simulink model "ModBateria"  (R2023a)
settings: Solver=VariableStepAuto  StartTime=0.0  StopTime=3600  RelTol=1e-3  AbsTol=1e-3  EnableMultiTasking=on
libraries: fl_lib x6, nesl_utility x5, batteryecm_lib x1
settings Model: Creator=Julian  LastModifiedBy=Julian
settings SolverCC: AutoScaleAbsTol=off  AlgebraicLoopSolver=TrustRegion  MaxZcPerStep=1
settings DataIOCC: LimitDataPoints=on  MaxDataPoints=10000
settings OptimizationCC: ReuseModelBlockBuffer=off  LifeSpan=inf
settings DebuggingCC: UnconnectedInputMsg=warning  UnconnectedOutputMsg=warning  UnconnectedLineMsg=warning  AllowSymbolicDim=off  SFUnexpectedBacktrackingDiag=warning  SFNoUnconditionalDefaultTransitionDiag=warning  SFExecutionAtInitializationDiag=none  ArithmeticOperatorsInVariantConditions=warning
settings ModelReferenceCC: EnableRefExpFcnMdlSchedulingChecks=on
settings SFSimCC: SimUseLocalCustomCode=off  CustomCodeUndefinedFunction=UseInterfaceOnly
settings RTWCC: RTWUseLocalCustomCode=off  DLArmComputeVersion=19.05
settings CodeAppCC: StateflowObjectComments=on
settings GRTTargetCC: TargetLangStandard=C89/C90 (ANSI)
settings ConfigComp: CovMetricSettings=dw  CovSaveCumulativeToWorkspaceVar=on  CovSaveSingleToWorkspaceVar=on  CovExternalEMLEnable=off  CovSFcnEnable=off
settings SimscapeCC: SimscapeLogType=all  SimscapeLogSimulationStatistics=on  SimscapeLogDataHistory=10000

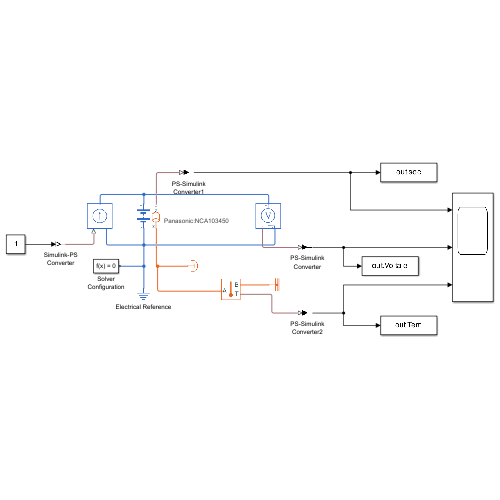
[thumbnail: Simulink's stored preview of the top-level diagram]
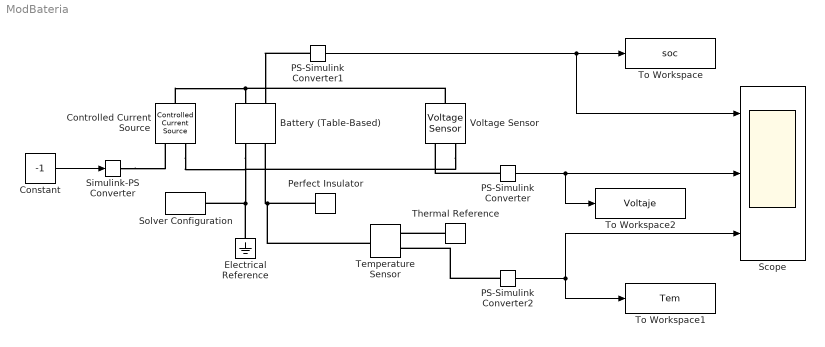
== system ModBateria ==
  Battery (Table-Based) : batteryecm_lib/Battery (Table-Based)  Tag={'toolbox/physmod/battery/shared_library/m/batteryecm_lib_parts';'Battery__Table_Based_/Panasonic/NCA103450.xml'}  SOC_vec=[0 0.01 0.02 0.03 0.04 0.05 0.06 0.07 0.08 0.09 0.1 0.11 0.12 0.13 0.14 0.15 0.16 0.17 0.18 0.19 0.2 0.21 0.22 0.23 0.24 0.25 0.26 0.27 0.28 0.29 0.3 0.31 0.32 0.33 0.34 0.35 0.36 0.37 0.38 0.39 0.4 0.41 0.42 0.43 0.44 0.45 0.46 0.47 0.48 0.49 0.5 0.51 0.52 0.53 0.54 0.55 0.56 0.57 0.58 0.59 0.6 0.61 0.62 0.63 0.64 0.65 0.66 0.67 0.68 0.69 0.7 0.71 0.72 0.73 0.74 0.75 0.76 0.77 0.78 0.79 0.8 0.81 0.82 0.83 0.84 0.85 0.86 0.87 0.88 0.89 0.9 0.91 0.92 0.93 0.94 0.95 0.96 0.97 0.98 0.99 1]  T_dependence=simscape.enum.tablebattery.temperature_dependence.yes  prm_dir=simscape.enum.tablebattery.prm_dir.noCurrentDirectionality  T_vec=[-20 -10 0 25 40] degC  V0_mat=[2.78866 2.78866 2.78866 2.78866 2.78866;2.85705 2.85705 2.85705 2.85705 2.85705;2.9399 2.9399 2.9399 2.9399 2.9399;2.9762 2.9762 2.9762 2.9762 2.9762;3.01251 3.01251 3.01251 3.01251 3.01251;3.04882 3.04882 3.04882 3.04882 3.04882;3.10085 3.10085 3.10085 3.10085 3.10085;3.15288 3.15288 3.15288 3.15288 3.15288;3.19526 3.19526 3.19526 3.19526 3.19526;3.23378 3.23378 3.23378 3.23378 3.23378;3.27026 3.27026 3.27026 3.27026 3.27026;3.29683 3.29683 3.29683 3.29683 3.29683;3.3202 3.3202 3.3202 3.3202 3.3202;3.34216 3.34216 3.34216 3.34216 3.34216;3.36071 3.36071 3.36071 3.36071 3.36071;3.37869 3.37869 3.37869 3.37869 3.37869;3.39522 3.39522 3.39522 3.39522 3.39522;3.40936 3.40936 3.40936 3.40936 3.40936;3.42116 3.42116 3.42116 3.42116 3.42116;3.43247 3.43247 3.43247 3.43247 3.43247;3.44296 3.44296 3.44296 3.44296 3.44296;3.45253 3.45253 3.45253 3.45253 3.45253;3.4621 3.4621 3.4621 3.4621 3.4621;3.47168 3.47168 3.47168 3.47168 3.47168;3.47981 3.47981 3.47981 3.47981 3.47981;3.48589 3.48589 3.48589 3.48589 3.48589;3.49191 3.49191 3.49191 3.49191 3.49191;3.49852 3.49852 3.49852 3.49852 3.49852;3.50514 3.50514 3.50514 3.50514 3.50514;3.51166 3.51166 3.51166 3.51166 3.51166;3.51793 3.51793 3.51793 3.51793 3.51793;3.52413 3.52413 3.52413 3.52413 3.52413;3.53014 3.53014 3.53014 3.53014 3.53014;3.5361 3.5361 3.5361 3.5361 3.5361;3.5422 3.5422 3.5422 3.5422 3.5422;3.5486 3.5486 3.5486 3.5486 3.5486;3.55501 3.55501 3.55501 3.55501 3.55501;3.56135 3.56135 3.56135 3.56135 3.56135;3.56757 3.56757 3.56757 3.56757 3.56757;3.57378 3.57378 3.57378 3.57378 3.57378;3.5802 3.5802 3.5802 3.5802 3.5802;3.58658 3.58658 3.58658 3.58658 3.58658;3.59285 3.59285 3.59285 3.59285 3.59285;3.59911 3.59911 3.59911 3.59911 3.59911;3.60522 3.60522 3.60522 3.60522 3.60522;3.61126 3.61126 3.61126 3.61126 3.61126;3.6173 3.6173 3.6173 3.6173 3.6173;3.62334 3.62334 3.62334 3.62334 3.62334;3.62937 3.62937 3.62937 3.62937 3.62937;3.63541 3.63541 3.63541 3.63541 3.63541;3.64172 3.64172 3.64172 3.64172 3.64172;3.65002 3.65002 3.65002 3.65002 3.65002;3.65922 3.65922 3.65922 3.65922 3.65922;3.66843 3.66843 3.66843 3.66843 3.66843;3.67774 3.67774 3.67774 3.67774 3.67774;3.68705 3.68705 3.68705 3.68705 3.68705;3.69636 3.69636 3.69636 3.69636 3.69636;3.70567 3.70567 3.70567 3.70567 3.70567;3.71498 3.71498 3.71498 3.71498 3.71498;3.72395 3.72395 3.72395 3.72395 3.72395;3.73263 3.73263 3.73263 3.73263 3.73263;3.74129 3.74129 3.74129 3.74129 3.74129;3.74974 3.74974 3.74974 3.74974 3.74974;3.75815 3.75815 3.75815 3.75815 3.75815;3.76656 3.76656 3.76656 3.76656 3.76656;3.77497 3.77497 3.77497 3.77497 3.77497;3.78345 3.78345 3.78345 3.78345 3.78345;3.79201 3.79201 3.79201 3.79201 3.79201;3.80058 3.80058 3.80058 3.80058 3.80058;3.80915 3.80915 3.80915 3.80915 3.80915;3.81772 3.81772 3.81772 3.81772 3.81772;3.8263 3.8263 3.8263 3.8263 3.8263;3.83493 3.83493 3.83493 3.83493 3.83493;3.84366 3.84366 3.84366 3.84366 3.84366;3.8525 3.8525 3.8525 3.8525 3.8525;3.86255 3.86255 3.86255 3.86255 3.86255;3.87289 3.87289 3.87289 3.87289 3.87289;3.88332 3.88332 3.88332 3.88332 3.88332;3.89375 3.89375 3.89375 3.89375 3.89375;3.90419 3.90419 3.90419 3.90419 3.90419;3.91462 3.91462 3.91462 3.91462 3.91462;3.92505 3.92505 3.92505 3.92505 3.92505;3.93549 3.93549 3.93549 3.93549 3.93549;3.9468 3.9468 3.9468 3.9468 3.9468;3.95849 3.95849 3.95849 3.95849 3.95849;3.97034 3.97034 3.97034 3.97034 3.97034;3.98295 3.98295 3.98295 3.98295 3.98295;3.99562 3.99562 3.99562 3.99562 3.99562;4.0083 4.0083 4.0083 4.0083 4.0083;4.02097 4.02097 4.02097 4.02097 4.02097;4.03332 4.03332 4.03332 4.03332 4.03332;4.04495 4.04495 4.04495 4.04495 4.04495;4.05596 4.05596 4.05596 4.05596 4.05596;4.06698 4.06698 4.06698 4.06698 4.06698;4.0778 4.0778 4.0778 4.0778 4.0778;4.0887 4.0887 4.0887 4.0887 4.0887;4.10062 4.10062 4.10062 4.10062 4.10062;4.11408 4.11408 4.11408 4.11408 4.11408;4.12548 4.12548 4.12548 4.12548 4.12548;4.13345 4.13345 4.13345 4.13345 4.13345;4.05294 4.05294 4.05294 4.05294 4.05294] V  V0_vec=[2.78866 2.85705 2.9399 2.9762 3.01251 3.04882 3.10085 3.15288 3.19526 3.23378 3.27026 3.29683 3.3202 3.34216 3.36071 3.37869 3.39522 3.40936 3.42116 3.43247 3.44296 3.45253 3.4621 3.47168 3.47981 3.48589 3.49191 3.49852 3.50514 3.51166 3.51793 3.52413 3.53014 3.5361 3.5422 3.5486 3.55501 3.56135 3.56757 3.57378 3.5802 3.58658 3.59285 3.59911 3.60522 3.61126 3.6173 3.62334 3.62937 3.63541 3.64172 3.65002 3.65922 3.66843 3.67774 3.68705 3.69636 3.70567 3.71498 3.72395 3.73263 3.74129 3.74974 3.75815 3.76656 3.77497 3.78345 3.79201 3.80058 3.80915 3.81772 3.8263 3.83493 3.84366 3.8525 3.86255 3.87289 3.88332 3.89375 3.90419 3.91462 3.92505 3.93549 3.9468 3.95849 3.97034 3.98295 3.99562 4.0083 4.02097 4.03332 4.04495 4.05596 4.06698 4.0778 4.0887 4.10062 4.11408 4.12548 4.13345 4.05294] V  V_range=[2.475 Inf] V  R0_mat=[0.53219 0.30004 0.37039 0.09603 0.02438;0.53219 0.49271 0.49416 0.09983 0.00588;0.53219 0.4834 0.47641 0.10832 0.00588;0.53219 0.47409 0.45867 0.10252 0.00588;0.53219 0.46477 0.44092 0.09675 0.00588;0.53219 0.45546 0.42317 0.09122 0.00588;0.53219 0.44615 0.40543 0.09227 0.01303;0.53219 0.43683 0.38768 0.09475 0.02948;0.53219 0.42752 0.36993 0.09603 0.04205;0.53219 0.4182 0.35219 0.09767 0.05287;0.53219 0.40889 0.33444 0.10033 0.06277;0.53219 0.39958 0.31669 0.10063 0.06815;0.53219 0.39026 0.29895 0.10093 0.07208;0.53219 0.38095 0.2812 0.10152 0.07537;0.53219 0.37164 0.26345 0.10164 0.07711;0.53219 0.36232 0.24546 0.10179 0.0786;0.52242 0.35301 0.22688 0.10206 0.081;0.51265 0.3437 0.2212 0.1018 0.0832;0.50288 0.33438 0.21445 0.10114 0.08432;0.49311 0.32507 0.20748 0.101 0.08523;0.48334 0.31575 0.20014 0.10083 0.08577;0.47357 0.30603 0.19554 0.10046 0.08589;0.4638 0.29631 0.19194 0.1001 0.086;0.45402 0.28659 0.18835 0.09973 0.08612;0.44425 0.27918 0.1841 0.09895 0.08559;0.43448 0.27108 0.17892 0.09787 0.08412;0.42471 0.26296 0.17371 0.09686 0.08262;0.41494 0.2551 0.16877 0.0964 0.08139;0.40517 0.24775 0.16605 0.09595 0.08017;0.3954 0.2429 0.16407 0.09547 0.07932;0.38563 0.23793 0.16198 0.09493 0.07894;0.37586 0.23293 0.15986 0.09438 0.07852;0.36609 0.22784 0.15765 0.09383 0.07801;0.35632 0.22273 0.15542 0.09328 0.07749;0.34661 0.21769 0.15325 0.09286 0.07702;0.33705 0.21414 0.15123 0.09268 0.0767;0.32749 0.2112 0.1492 0.0925 0.07637;0.31951 0.20824 0.14714 0.0923 0.07602;0.31183 0.20521 0.14536 0.09207 0.07561;0.30415 0.20219 0.14439 0.09183 0.0752;0.29737 0.19925 0.1435 0.09158 0.07488;0.29162 0.19631 0.14261 0.09129 0.07454;0.28581 0.1933 0.14165 0.09097 0.07415;0.28 0.19104 0.1407 0.09065 0.07376;0.27413 0.18925 0.13968 0.09019 0.07331;0.26997 0.18743 0.13863 0.08966 0.07252;0.26679 0.18561 0.13757 0.08913 0.07134;0.26361 0.18379 0.13652 0.0886 0.07015;0.26043 0.18196 0.13546 0.08807 0.06897;0.25726 0.18014 0.13423 0.08754 0.06779;0.2542 0.17844 0.13297 0.08709 0.06673;0.25206 0.17765 0.13261 0.08715 0.06658;0.25091 0.17727 0.13266 0.08735 0.06684;0.24985 0.17693 0.13272 0.08754 0.0671;0.24884 0.1769 0.13282 0.08783 0.0674;0.24782 0.17687 0.13292 0.08812 0.06771;0.24681 0.17684 0.13302 0.08841 0.06802;0.2458 0.17681 0.13312 0.08871 0.06832;0.24487 0.17678 0.13322 0.089 0.06863;0.24411 0.17659 0.13316 0.08898 0.06878;0.2432 0.17627 0.13298 0.08885 0.0688;0.24229 0.17595 0.13278 0.08873 0.06881;0.24128 0.17552 0.13249 0.08856 0.06873;0.24026 0.17508 0.13264 0.08838 0.06862;0.23923 0.17486 0.13281 0.0882 0.06852;0.23835 0.17524 0.13297 0.08802 0.06831;0.23811 0.17565 0.13317 0.0879 0.06809;0.23791 0.17609 0.1334 0.08786 0.0679;0.23771 0.17654 0.13364 0.08782 0.06772;0.23751 0.17699 0.13388 0.08777 0.06753;0.23731 0.17744 0.13412 0.08773 0.06735;0.23712 0.17789 0.13435 0.08769 0.06717;0.23776 0.17838 0.13462 0.08766 0.06701;0.23888 0.1789 0.13493 0.08765 0.0669;0.24006 0.17947 0.13529 0.08775 0.06684;0.24178 0.18059 0.1362 0.08831 0.06733;0.24363 0.18296 0.13773 0.08891 0.06795;0.24612 0.18543 0.13994 0.0895 0.06861;0.24943 0.18789 0.14215 0.09009 0.06927;0.25274 0.19036 0.14435 0.09068 0.06994;0.25605 0.19282 0.14656 0.09128 0.0706;0.25936 0.19528 0.14877 0.09187 0.07061;0.26267 0.19775 0.15098 0.09246 0.07051;0.26675 0.20061 0.15359 0.09325 0.07081;0.27411 0.20718 0.15638 0.09414 0.07128;0.28153 0.21446 0.15923 0.09506 0.07182;0.2893 0.22209 0.16243 0.09659 0.0727;0.29711 0.22975 0.16671 0.09819 0.07362;0.3107 0.23741 0.17308 0.09978 0.07454;0.3255 0.24641 0.17945 0.10137 0.07546;0.34015 0.25878 0.18568 0.10289 0.07623;0.35449 0.27083 0.19158 0.10428 0.07667;0.37901 0.2826 0.19719 0.10573 0.07611;0.40352 0.29437 0.20281 0.10718 0.07533;0.43288 0.30464 0.20866 0.10844 0.07446;0.46442 0.31432 0.21473 0.10966 0.07362;0.48999 0.32446 0.22126 0.1111 0.07325;0.50843 0.33529 0.22849 0.11285 0.07358;0.51485 0.3452 0.22623 0.11028 0.07297;0.50978 0.33242 0.2214 0.10452 0.0708;0.43991 0.2781 0.17636 0.0168 0.02841] Ohm  R0_vec=[0.09603 0.09983 0.10832 0.10252 0.09675 0.09122 0.09227 0.09475 0.09603 0.09767 0.10033 0.10063 0.10093 0.10152 0.10164 0.10179 0.10206 0.1018 0.10114 0.101 0.10083 0.10046 0.1001 0.09973 0.09895 0.09787 0.09686 0.0964 0.09595 0.09547 0.09493 0.09438 0.09383 0.09328 0.09286 0.09268 0.0925 0.0923 0.09207 0.09183 0.09158 0.09129 0.09097 0.09065 0.09019 0.08966 0.08913 0.0886 0.08807 0.08754 0.08709 0.08715 0.08735 0.08754 0.08783 0.08812 0.08841 0.08871 0.089 0.08898 0.08885 0.08873 0.08856 0.08838 0.0882 0.08802 0.0879 0.08786 0.08782 0.08777 0.08773 0.08769 0.08766 0.08765 0.08775 0.08831 0.08891 0.0895 0.09009 0.09068 0.09128 0.09187 0.09246 0.09325 0.09414 0.09506 0.09659 0.09819 0.09978 0.10137 0.10289 0.10428 0.10573 0.10718 0.10844 0.10966 0.1111 0.11285 0.11028 0.10452 0.0168] Ohm  R0_dis_mat=[.0117, .0085, .009; .011, .0085, .009; .0114, .0087, .0092; .0107, .0082, .0088; .0107, .0083, .0091; .0113, .0085, .0089; .0116, .0085, .0089] % Parameter not set Ohm  R0_dis_vec=[.0085, .0085, .0087, .0082, .0083, .0085, .0085] % Parameter not set Ohm  R0_ch_mat=[.0117, .0085, .009; .011, .0085, .009; .0114, .0087, .0092; .0107, .0082, .0088; .0107, .0083, .0091; .0113, .0085, .0089; .0116, .0085, .0089] % Parameter not set Ohm  R0_ch_vec=[.0085, .0085, .0087, .0082, .0083, .0085, .0085] % Parameter not set Ohm  AH=2.318 hr*A  prm_leak=simscape.enum.tablebattery.prm_leak.disabled  Rleak_vec=[8000, 7000, 6000] % Parameter not set Ohm  Rleak=7e3 % Parameter not set Ohm  extrapolation_option=simscape.enum.extrapolation.nearest  SOC_port=simscape.enum.tablebattery.enable.yes  prm_dyn=simscape.enum.tablebattery.prm_dyn.off  R1_mat=[.0109, .0029, .0013; .0069, .0024, .0012; .0047, .0026, .0013; .0034, .0016, .001; .0033, .0023, .0014; .0033, .0018, .0011; .0028, .0017, .0011] % Parameter not set Ohm  R1_vec=[.0029, .0024, .0026, .0016, .0023, .0018, .0017] % Parameter not set Ohm  tau1_mat=[20, 36, 39; 31, 45, 39; 109, 105, 61; 36, 29, 26; 59, 77, 67; 40, 33, 29; 25, 39, 33] % Parameter not set s  tau1_vec=[36, 45, 105, 29, 77, 33, 39] % Parameter not set s  R2_mat=[.0109, .0029, .0013; .0069, .0024, .0012; .0047, .0026, .0013; .0034, .0016, .001; .0033, .0023, .0014; .0033, .0018, .0011; .0028, .0017, .0011] % Parameter not set Ohm  R2_vec=[.0029, .0024, .0026, .0016, .0023, .0018, .0017] % Parameter not set Ohm  tau2_mat=[20, 36, 39; 31, 45, 39; 109, 105, 61; 36, 29, 26; 59, 77, 67; 40, 33, 29; 25, 39, 33] % Parameter not set s  tau2_vec=[36, 45, 105, 29, 77, 33, 39] % Parameter not set s  R3_mat=[.0109, .0029, .0013; .0069, .0024, .0012; .0047, .0026, .0013; .0034, .0016, .001; .0033, .0023, .0014; .0033, .0018, .0011; .0028, .0017, .0011] % Parameter not set Ohm  R3_vec=[.0029, .0024, .0026, .0016, .0023, .0018, .0017] % Parameter not set Ohm  tau3_mat=[20, 36, 39; 31, 45, 39; 109, 105, 61; 36, 29, 26; 59, 77, 67; 40, 33, 29; 25, 39, 33] % Parameter not set s  tau3_vec=[36, 45, 105, 29, 77, 33, 39] % Parameter not set s  R4_mat=[.0109, .0029, .0013; .0069, .0024, .0012; .0047, .0026, .0013; .0034, .0016, .001; .0033, .0023, .0014; .0033, .0018, .0011; .0028, .0017, .0011] % Parameter not set Ohm  R4_vec=[.0029, .0024, .0026, .0016, .0023, .0018, .0017] % Parameter not set Ohm  tau4_mat=[20, 36, 39; 31, 45, 39; 109, 105, 61; 36, 29, 26; 59, 77, 67; 40, 33, 29; 25, 39, 33] % Parameter not set s  tau4_vec=[36, 45, 105, 29, 77, 33, 39] % Parameter not set s  R5_mat=[.0109, .0029, .0013; .0069, .0024, .0012; .0047, .0026, .0013; .0034, .0016, .001; .0033, .0023, .0014; .0033, .0018, .0011; .0028, .0017, .0011] % Parameter not set Ohm  R5_vec=[.0029, .0024, .0026, .0016, .0023, .0018, .0017] % Parameter not set Ohm  tau5_mat=[20, 36, 39; 31, 45, 39; 109, 105, 61; 36, 29, 26; 59, 77, 67; 40, 33, 29; 25, 39, 33] % Parameter not set s  tau5_vec=[36, 45, 105, 29, 77, 33, 39] % Parameter not set s  prm_fade=simscape.enum.tablebattery.prm_fade.tableN  N0=100 % Parameter not set  dV0=0 % Parameter not set  dR0=0 % Parameter not set  dAH=0 % Parameter not set  dRleak=0 % Parameter not set  dR1=0 % Parameter not set  dR2=0 % Parameter not set  dR3=0 % Parameter not set  dR4=0 % Parameter not set  dR5=0 % Parameter not set  N0vec=[1 6 11 16 21 26 31 36 41 46 51 56 61 66 71 76 81 86 91 96 101 106 111 116 121 126 131 136 141 146 151 156 161 166 171 176 181 186 191 196 201 206 211 216 221 226 231 236 241 246 251 256 261 266 271 276 281 286 291 296 301 306 311 316 321 326 331 336 341 346 351 356 361 366 371 376 381 386 391 396 401 406 411 416 421 426 431 436 441 446 451 456 461 466 471 476 481 486 491 496]  Tfadevec=[298.15, 323.15] % Parameter not set K  dV0vec=[0 1.1011 1.9651 1.8561 1.7287 1.5728 1.5093 1.4645 1.4195 1.3746 1.3297 1.2848 1.2398 1.1949 1.153 1.1132 1.0701 1.0189 0.9677 0.9164 0.8667 0.8198 0.7729 0.726 0.6792 0.6323 0.5856 0.5391 0.4926 0.4462 0.4085 0.3715 0.3343 0.2966 0.2589 0.2212 0.1836 0.1459 0.1082 0.0706 0.0329 -0.0048 -0.0425 -0.0801 -0.1178 -0.1452 -0.1645 -0.1838 -0.2035 -0.2238 -0.2442 -0.2646 -0.285 -0.3053 -0.3257 -0.3461 -0.3664 -0.3868 -0.4072 -0.43 -0.4664 -0.504 -0.5427 -0.5813 -0.62 -0.6587 -0.6974 -0.7361 -0.7748 -0.8141 -0.8538 -0.8935 -0.9332 -0.9705 -0.9993 -1.0281 -1.0569 -1.0857 -1.1145 -1.1433 -1.1721 -1.2009 -1.2297 -1.2585 -1.2873 -1.3161 -1.3447 -1.3602 -1.3757 -1.3912 -1.4068 -1.4223 -1.4378 -1.4533 -1.4688 -1.4843 -1.4998 -1.5153 -1.5308 -1.5463]  dR0vec=[0 0 0 0 0 0 0 0 0 0 0 0 0 0 0 0 0 0 0 0 0 0 0 0 0 0 0 0 0 0 0 0 0 0 0 0 0 0 0 0 0 0 0 0 0 0 0 0 0 0 0 0 0 0 0 0 0 0 0 0 0 0 0 0 0 0 0 0 0 0 0 0 0 0 0 0 0 0 0 0 0 0 0 0 0 0 0 0 0 0 0 0 0 0 0 0 0 0 0 0] % Parameter assumed  dAHvec=[0 -0.554 -1.109 -1.663 -2.217 -2.772 -2.997 -3.133 -3.268 -3.403 -3.539 -3.674 -3.809 -3.945 -4.08 -4.215 -4.362 -4.536 -4.71 -4.885 -5.059 -5.233 -5.407 -5.581 -5.755 -5.93 -6.104 -6.278 -6.452 -6.626 -6.768 -6.906 -7.045 -7.183 -7.322 -7.461 -7.599 -7.738 -7.876 -8.015 -8.154 -8.292 -8.431 -8.57 -8.708 -8.809 -8.88 -8.951 -9.022 -9.093 -9.164 -9.235 -9.306 -9.377 -9.448 -9.519 -9.59 -9.661 -9.732 -9.812 -9.939 -10.066 -10.192 -10.319 -10.446 -10.573 -10.7 -10.827 -10.954 -11.081 -11.208 -11.335 -11.462 -11.581 -11.673 -11.766 -11.858 -11.95 -12.042 -12.134 -12.226 -12.318 -12.41 -12.502 -12.594 -12.686 -12.778 -12.828 -12.877 -12.927 -12.976 -13.026 -13.076 -13.125 -13.175 -13.224 -13.274 -13.323 -13.373 -13.423]  dRleakvec=[0, 0, 0] % Parameter not set  dR1vec=[0, 0, 0] % Parameter not set  dR2vec=[0, 0, 0] % Parameter not set  dR3vec=[0, 0, 0] % Parameter not set  dR4vec=[0, 0, 0] % Parameter not set  dR5vec=[0, 0, 0] % Parameter not set  dV0mat=[0, 0; 0, 0; 0, 0] % Parameter not set  dR0mat=[0, 0; 0, 0; 0, 0] % Parameter not set  dAHmat=[0, 0; 0, 0; 0, 0] % Parameter not set  dRleakmat=[0, 0; 0, 0; 0, 0] % Parameter not set  dR1mat=[0, 0; 0, 0; 0, 0] % Parameter not set  dR2mat=[0, 0; 0, 0; 0, 0] % Parameter not set  dR3mat=[0, 0; 0, 0; 0, 0] % Parameter not set  dR4mat=[0, 0; 0, 0; 0, 0] % Parameter not set  dR5mat=[0, 0; 0, 0; 0, 0] % Parameter not set  prm_age_modeling=simscape.enum.tablebattery.prm_age_modeling.equation  storage_dt_age_vec=[0] % Parameter not set d  storage_T_age_vec=[273] % Parameter not set K  prm_age_OCV=simscape.enum.tablebattery.prm_age_OCV.OCV  OCV_age=0.9 % Parameter not set  SOC_age=0.6 % Parameter not set  prm_age_resistance=simscape.enum.tablebattery.prm_age.disabled  OCV_scaling_age_resistance=2.2134e6 % Parameter not set  OCV_offset_age_resistance=1.632e6 % Parameter not set  temp_exp_age_resistance=0.515833569 % Parameter not set V  t_exp_age_resistance=0.75 % Parameter not set  T_age_vec_resistance=[273.15, 298.15, 323.15] % Parameter not set K  dt_age_vec_resistance=[90, 180, 270, 360] % Parameter not set d  dR0_age_vec=[0, 0, 0] % Parameter not set  t_meas_dR0_age=100 % Parameter not set d  dR0_age_mat=[0, 0, 0; 0, 0, 0; 0, 0, 0; 0, 0, 0] % Parameter not set  prm_age_capacity=simscape.enum.tablebattery.prm_age.disabled  OCV_scaling_age_capacity=1.5097e07 % Parameter not set  OCV_offset_age_capacity=8.3625e06 % Parameter not set  temp_exp_age_capacity=0.6011 % Parameter not set V  t_exp_age_capacity=0.75 % Parameter not set  T_age_vec_capacity=[273.15, 298.15, 323.15] % Parameter not set K  dt_age_vec_capacity=[90, 180, 270, 360] % Parameter not set d  dAH_age_vec=[0, 0, 0] % Parameter not set  t_meas_dAH_age=100 % Parameter not set d  dAH_age_mat=[0, 0, 0; 0, 0, 0; 0, 0, 0; 0, 0, 0] % Parameter not set  thermal_port=simscape.enum.thermaleffects.model  temperature=298.15 % Parameter not set K  thermal_mass=34.47 % Parameter assumed J/K  i_specify=off  i_priority=None  i=0 A  i_nominal_specify=off  i_nominal_unit=A  i_nominal_value=1  v_specify=off  v_priority=None  v=0 V  v_nominal_specify=off  v_nominal_unit=V  v_nominal_value=1  stateOfCharge_specify=off  stateOfCharge_priority=High  stateOfCharge=1  stateOfCharge_nominal_specify=off  stateOfCharge_nominal_unit=1  stateOfCharge_nominal_value=1  num_cycles_specify=off  num_cycles_priority=High  num_cycles=0  num_cycles_nominal_specify=off  num_cycles_nominal_unit=1  num_cycles_nominal_value=1  cell_temperature_specify=off  cell_temperature_priority=High  cell_temperature=298.15 K  cell_temperature_nominal_specify=off  cell_temperature_nominal_unit=K  cell_temperature_nominal_value=1
      settings: AttributesFormatString=Panasonic:NCA103450
  Constant : Constant  Value=-1
  Controlled Current Source : fl_lib/Electrical/Electrical Sources/Controlled Current Source
  Electrical Reference : fl_lib/Electrical/Electrical Elements/Electrical Reference
  PS-Simulink Converter : nesl_utility/PS-Simulink Converter  PhysicalDomain=network_engine_domain  SubClassName=ps_output  LeftPortType=input  RightPortType=output  PseudoPeriodic=off  Frequencies=[]  VectorFormat=inherit  Unit=inherit  AffineConversion=off
  PS-Simulink Converter1 : nesl_utility/PS-Simulink Converter  PhysicalDomain=network_engine_domain  SubClassName=ps_output  LeftPortType=input  RightPortType=output  PseudoPeriodic=off  Frequencies=[]  VectorFormat=inherit  Unit=inherit  AffineConversion=off
  PS-Simulink Converter2 : nesl_utility/PS-Simulink Converter  PhysicalDomain=network_engine_domain  SubClassName=ps_output  LeftPortType=input  RightPortType=output  PseudoPeriodic=off  Frequencies=[]  VectorFormat=inherit  Unit=inherit  AffineConversion=off
  Perfect Insulator : fl_lib/Thermal/Thermal Elements/Perfect Insulator  T_specify=off  T_priority=None  T=293.15 K  T_nominal_specify=off  T_nominal_unit=K  T_nominal_value=1
  Scope : Scope  NumInputPorts=3
  Simulink-PS Converter : nesl_utility/Simulink-PS Converter  PhysicalDomain=network_engine_domain  SubClassName=ps_input  LeftPortType=input  RightPortType=output  PseudoPeriodic=off  Frequencies=[]  NoiseDistribution=none  NoiseParameters=[]  Unit=1  AffineConversion=off  FilteringAndDerivatives=provide  SimscapeFilterOrder=1  InputFilterTimeConstant=0.001  UdotUserProvided=0
  Solver Configuration : nesl_utility/Solver Configuration  PhysicalDomain=network_engine_domain  SubClassName=solver  LeftPortType=input  RightPortType=generic  Tones=[]  Harmonics=[]  SimulateNoise=off  Profile=off  UseLocalSampling=off  EnableSwitchedLinearOptims=on  FrequencyDomain=off  UseCCode=off  RelTol=0.001  AbsTol=1e-06  MinStep=1e-09  ToWorkspace=off  RevertToSquareIcSolve=off  NumHomotopyIterations=100  PhasorMode=off  PhasorModeNumHarmonics=1  ConsistencySolver=NEWTON_XTOL_AFTER_FTOL  IndexReductionMethod=DerivativeReplacement  DoDC=off  ResidualTolerance=1e-09  ConsistencyTolSource=GLOBAL  ConsistencyAbsTol=0.001  ConsistencyRelTol=0.001  ConsistencyTolFactor=0.001  UseLocalSolver=off  LocalSolverChoice=NE_BACKWARD_EULER_ADVANCER  ResolveIndetEquations=on  FunctionEvalNumThread=1  LocalSolverSampleTime=0.001  DoFixedCost=off  MaxNonlinIter=3  MaxModeIter=2  ComputeImpulses=off  ImpulseIterations=2  LinearAlgebra=auto  LinearAlgebraNumThread=0  EquationFormulation=NE_TIME_EF  DelaysMemoryBudget=1024  AutomaticFiltering=on  FilteringTimeConstant=0.001  PartitionStorageMethod=AS_NEEDED  PartitionMemoryBudget=1024  PartitionMethod=ROBUST
  Temperature Sensor : fl_lib/Thermal/Thermal Sensors/Temperature Sensor  temperature_measure=foundation.enum.MeasurementReference.difference
  Thermal Reference : fl_lib/Thermal/Thermal Elements/Thermal Reference
  To Workspace : ToWorkspace  VariableName=soc  SampleTime=-1
  To Workspace1 : ToWorkspace  VariableName=Tem  SampleTime=-1
  To Workspace2 : ToWorkspace  VariableName=Voltaje  SampleTime=-1
  Voltage Sensor : fl_lib/Electrical/Electrical Sensors/Voltage Sensor
  wires:
  PS-Simulink Converter/1 -> To Workspace2/1, Scope/2
  Constant/1 -> Simulink-PS Converter/1
  PS-Simulink Converter1/1 -> To Workspace/1, Scope/1
  PS-Simulink Converter2/1 -> To Workspace1/1, Scope/3
  connections:
  Electrical Reference/LConn1 -- Voltage Sensor/RConn2 -- Controlled Current Source/RConn2 -- Battery (Table-Based)/RConn1 -- Solver Configuration/RConn1
  Controlled Current Source/LConn1 -- Voltage Sensor/LConn1 -- Battery (Table-Based)/LConn1
  Perfect Insulator/LConn1 -- Temperature Sensor/LConn1 -- Battery (Table-Based)/RConn2
  Simulink-PS Converter/RConn1 -- Controlled Current Source/RConn1
  PS-Simulink Converter/LConn1 -- Voltage Sensor/RConn1
  PS-Simulink Converter1/LConn1 -- Battery (Table-Based)/LConn2
  Thermal Reference/LConn1 -- Temperature Sensor/RConn1
  PS-Simulink Converter2/LConn1 -- Temperature Sensor/RConn2
